simulink model "OpenClosedLoop"  (R2019a)
settings: Solver=VariableStepAuto  StartTime=0.0  StopTime=20.0  RelTol=1e-3
settings Model: Creator=G5  LastModifiedBy=G5

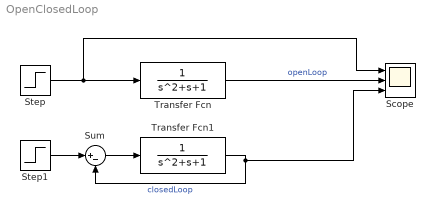
== system OpenClosedLoop ==
  Scope : Scope  NumInputPorts=3
  Step : Step  SampleTime=0
  Step1 : Step  SampleTime=0
  Sum : Sum  Inputs=|+-
  Transfer Fcn : TransferFcn  Denominator=[1 1 1]
  Transfer Fcn1 : TransferFcn  Denominator=[1 1 1]
  wires:
  Step/1 -> Scope/1, Transfer Fcn/1
  Transfer Fcn/1 -> Scope/2  "openLoop"
  Step1/1 -> Sum/1
  Sum/1 -> Transfer Fcn1/1
  Transfer Fcn1/1 -> Sum/2, Scope/3  "closedLoop"
